simulink model "Assignment2_6"  (R2021b)
settings: Solver=ode45  StartTime=0.0  StopTime=0.1  RelTol=1e-3
libraries: eeGeneralControl x12, spsGroundLib x6, spsSeriesRLCBranchLib x6, spsBreakerLib x5, spsCurrentMeasurementLib x4, spsSeriesRLCLoadLib x3, spsACVoltageSourceLib x2, spspowerguiLib x1
settings Model: Creator=yyx  LastModifiedBy=Divin

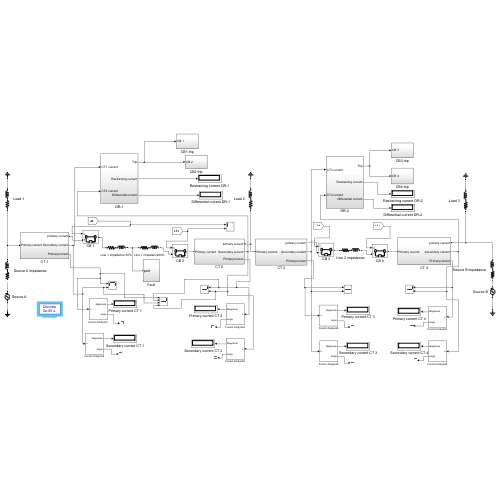
[thumbnail: Simulink's stored preview of the top-level diagram]
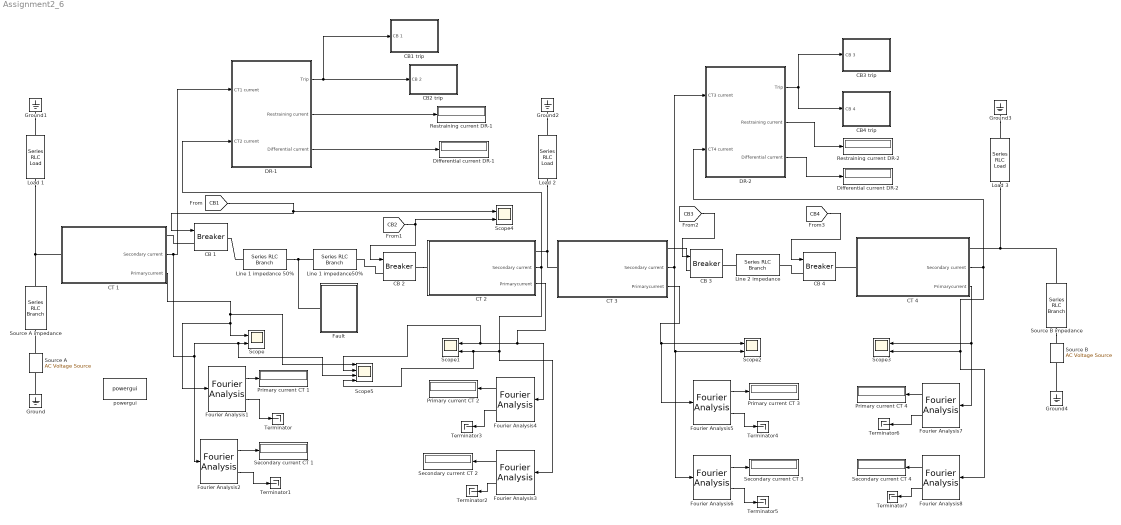
== system Assignment2_6 ==
  CB {1..4} (4 alike) : spsBreakerLib/Breaker  InitialState=1  SwitchingTimes="[1/60  5/60]"  External=on  BreakerResistance=0.01  SnubberResistance=1e6  SnubberCapacitance=inf  Measurements=None  MoreParameters=on  NoBreakLoop=off
      settings: SourceProductBaseCode=PS
  CB1 trip : Subsystem
  CB2 trip : Subsystem
  CB3 trip : Subsystem
  CB4 trip : Subsystem
  CT 1 : Subsystem
      settings: PortSchema="{\"entries\":[{\"content\":{\"sides\":[{\"content\":{\"connectorIds\":[\"LConn1\"]},\"type\":\"ConnectorPlacement.EquallySpacedRectSide\",\"uuid\":\"b6c390a4-07fb-4b4f-8c93-5dabcb0efae7\"},{\"content\":{\"connectorIds\":[\"RConn1\",\"Out1\",\"Out2\"],\"side\":\"RIGHT\"},\"type\":\"ConnectorPlacement.EquallySpacedRectSide\",\"uuid\":\"a4be9a2e-9ce7-48b9-b5c8-de816166e0f8\"},{\"content\":{\"connectorIds\":[],\"side\":\"TOP\"},\"type\":\"ConnectorPlacement.EquallySpacedRectSide\",\"uuid\":\"65e6e7fb-be75-4aba-a80b-3e233021d29a\"},{\"content\":{\"connectorIds\":[],\"side\":\"BOTTOM\"},\"type\":\"ConnectorPlacement.EquallySpacedRectSide\",\"uuid\":\"e137e53f-9924-4e8e-9c53-452c54d47921\"}]},\"type\":\"ConnectorPlacement.EquallySpacedConnector\",\"uuid\":\"c098d5a2-c3b9-46e4-a182-de1093aeec0c\"}],\"packageUris\":[\"http://schema.mathworks.com/mf0/Connector/R2020b\"],\"version\":\"1.0\"}"
  CT 2 : Subsystem
      settings: PortSchema="{\"entries\":[{\"content\":{\"sides\":[{\"content\":{\"connectorIds\":[\"LConn1\"]},\"type\":\"ConnectorPlacement.EquallySpacedRectSide\",\"uuid\":\"b6c390a4-07fb-4b4f-8c93-5dabcb0efae7\"},{\"content\":{\"connectorIds\":[\"RConn1\",\"Out1\",\"Out2\"],\"side\":\"RIGHT\"},\"type\":\"ConnectorPlacement.EquallySpacedRectSide\",\"uuid\":\"a4be9a2e-9ce7-48b9-b5c8-de816166e0f8\"},{\"content\":{\"connectorIds\":[],\"side\":\"TOP\"},\"type\":\"ConnectorPlacement.EquallySpacedRectSide\",\"uuid\":\"65e6e7fb-be75-4aba-a80b-3e233021d29a\"}]},\"type\":\"ConnectorPlacement.EquallySpacedConnector\",\"uuid\":\"c098d5a2-c3b9-46e4-a182-de1093aeec0c\"}],\"packageUris\":[\"http://schema.mathworks.com/mf0/Connector/R2020b\"],\"version\":\"1.0\"}"
  CT 3 : Subsystem
      settings: PortSchema="{\"entries\":[{\"content\":{\"sides\":[{\"content\":{\"connectorIds\":[\"LConn1\"]},\"type\":\"ConnectorPlacement.EquallySpacedRectSide\",\"uuid\":\"b6c390a4-07fb-4b4f-8c93-5dabcb0efae7\"},{\"content\":{\"connectorIds\":[\"RConn1\",\"Out1\",\"Out2\"],\"side\":\"RIGHT\"},\"type\":\"ConnectorPlacement.EquallySpacedRectSide\",\"uuid\":\"a4be9a2e-9ce7-48b9-b5c8-de816166e0f8\"},{\"content\":{\"connectorIds\":[],\"side\":\"TOP\"},\"type\":\"ConnectorPlacement.EquallySpacedRectSide\",\"uuid\":\"65e6e7fb-be75-4aba-a80b-3e233021d29a\"}]},\"type\":\"ConnectorPlacement.EquallySpacedConnector\",\"uuid\":\"c098d5a2-c3b9-46e4-a182-de1093aeec0c\"}],\"packageUris\":[\"http://schema.mathworks.com/mf0/Connector/R2020b\"],\"version\":\"1.0\"}"
  CT 4 : Subsystem
      settings: PortSchema="{\"entries\":[{\"content\":{\"sides\":[{\"content\":{\"connectorIds\":[\"LConn1\"]},\"type\":\"ConnectorPlacement.EquallySpacedRectSide\",\"uuid\":\"b6c390a4-07fb-4b4f-8c93-5dabcb0efae7\"},{\"content\":{\"connectorIds\":[\"RConn1\",\"Out1\",\"Out2\"],\"side\":\"RIGHT\"},\"type\":\"ConnectorPlacement.EquallySpacedRectSide\",\"uuid\":\"a4be9a2e-9ce7-48b9-b5c8-de816166e0f8\"},{\"content\":{\"connectorIds\":[],\"side\":\"TOP\"},\"type\":\"ConnectorPlacement.EquallySpacedRectSide\",\"uuid\":\"65e6e7fb-be75-4aba-a80b-3e233021d29a\"},{\"content\":{\"connectorIds\":[],\"side\":\"BOTTOM\"},\"type\":\"ConnectorPlacement.EquallySpacedRectSide\",\"uuid\":\"ae0a5bc8-40b7-4a3b-a403-59123a5fd983\"}]},\"type\":\"ConnectorPlacement.EquallySpacedConnector\",\"uuid\":\"c098d5a2-c3b9-46e4-a182-de1093aeec0c\"}],\"packageUris\":[\"http://schema.mathworks.com/mf0/Connector/R2020b\"],\"version\":\"1.0\"}"
  DR-1 : Subsystem
  DR-2 : Subsystem
  Differential current DR-1 : Display
  Differential current DR-2 : Display
  Fault : Subsystem
  Fourier Analysis{1..8} (8 alike) : eeGeneralControl/Fourier Analysis  f=60  n=[1]  M0=0  Ph0=0  BufferSize=8192  Ts=0
      settings: SourceProductBaseCode=PS
  Ground{,1..4} (5 alike) : spsGroundLib/Ground  LConnTagsString=a
  Line 1 impedance 50% : spsSeriesRLCBranchLib/Series RLC Branch  LConnTagsString=__new0  RConnTagsString=__new0  BranchType=RL  Resistance=1  Inductance=0.026525  SetiL0=off  InitialCurrent=0  Capacitance=1e-6  Setx0=off  InitialVoltage=0  Measurements=None
  Line 1 impedance50% : spsSeriesRLCBranchLib/Series RLC Branch  LConnTagsString=__new0  RConnTagsString=__new0  BranchType=RL  Resistance=1  Inductance=0.026525  SetiL0=off  InitialCurrent=0  Capacitance=1e-6  Setx0=off  InitialVoltage=0  Measurements=None
  Line 2 impedance : spsSeriesRLCBranchLib/Series RLC Branch  LConnTagsString=__new0  RConnTagsString=__new0  BranchType=RL  Resistance=2  Inductance=0.05305  SetiL0=off  InitialCurrent=0  Capacitance=1e-6  Setx0=off  InitialVoltage=0  Measurements=None
  Load 1 : spsSeriesRLCLoadLib/Series RLC Load  LConnTagsString=a  RConnTagsString=__new0  NominalVoltage=138000  NominalFrequency=60  ActivePower=100e6  InductivePower=30e6  CapacitivePower=0  Setx0=off  InitialVoltage=0  SetiL0=off  InitialCurrent=0  Measurements=None  LoadType=constant Z
  Load 2 : spsSeriesRLCLoadLib/Series RLC Load  LConnTagsString=a  RConnTagsString=__new0  NominalVoltage=138000  NominalFrequency=60  ActivePower=100e6  InductivePower=30e6  CapacitivePower=0  Setx0=off  InitialVoltage=0  SetiL0=off  InitialCurrent=0  Measurements=None  LoadType=constant Z
  Load 3 : spsSeriesRLCLoadLib/Series RLC Load  LConnTagsString=a  RConnTagsString=__new0  NominalVoltage=138000  NominalFrequency=60  ActivePower=100e6  InductivePower=30e6  CapacitivePower=0  Setx0=off  InitialVoltage=0  SetiL0=off  InitialCurrent=0  Measurements=None  LoadType=constant Z
  Primary current CT {1..4} (4 alike) : Display
  Restraining current DR-1 : Display
  Restraining current DR-2 : Display
  Scope{,1..4} (5 alike) : Scope  NumInputPorts=2
  Scope5 : Scope  NumInputPorts=4
  Secondary current CT {1..4} (4 alike) : Display
  Source A : spsACVoltageSourceLib/AC Voltage Source  Amplitude=158000  Phase=0  Frequency=60  SampleTime=0  Measurements=None  BusType=swing  Pref=10e3  Qref=0  Qmin=-inf  Qmax=+inf
  Source A impedance : spsSeriesRLCBranchLib/Series RLC Branch  LConnTagsString=__new0  RConnTagsString=__new0  BranchType=RL  Resistance=1  Inductance=0.02653  SetiL0=off  InitialCurrent=0  Capacitance=1e-6  Setx0=off  InitialVoltage=0  Measurements=None
  Source B : spsACVoltageSourceLib/AC Voltage Source  Amplitude=157000  Phase=-15  Frequency=60  SampleTime=0  Measurements=None  BusType=swing  Pref=10e3  Qref=0  Qmin=-inf  Qmax=+inf
  Source B impedance : spsSeriesRLCBranchLib/Series RLC Branch  LConnTagsString=__new0  RConnTagsString=__new0  BranchType=RL  Resistance=1  Inductance=0.02653  SetiL0=off  InitialCurrent=0  Capacitance=1e-6  Setx0=off  InitialVoltage=0  Measurements=None
  Terminator{,1..7} (8 alike) : Terminator
  powergui : spspowerguiLib/powergui  Priority=1  SimulationMode=Discrete  SampleTime=50e-6  frequency=60  Iterations=50  frequencyindice=0  Pbase=100e6  ErrMax=1e-4  UnitsV=kV  UnitsW=MW  buscounter=0  FunctionMessages=off  echomessages=off  EnableUseOfTLC=off  CurrentSourceSwitches=off  DisableSnubberDevices=off  DisableRonSwitches=off  DisableVfSwitches=off  DisplayEquations=off  AutomaticDiscreteSolvers=off  SolverType=Tustin/Backward Euler (TBE)  Interpol=off  ExternalGateDelay=off  methode=off  Ts=100  x0status=blocks  SPID=on  SwTol=0  HookPort=off  NonlinearTolerance=1e-4  nMaxIteration=100  ContinueOnMaxIteration=off  RestoreLinks=warning  ResistiveCurrentMeasurement=off  Frange=[0:2:500]  Ylog=off  Xlog=on  ShowGrid=off  save=off  variable=ZData  structure=0  ZoomFFT=off  StartTime=0.0  cycles=1  DisplayStyle=1  fundamental=60  FreqAxis=off  MaxFrequency=1000  frequencyindicesteady=1  RmsSteady=1  display=off
  wires:
  CT 2/1(Secondary current) -> Fourier Analysis3/1, Scope5/4, Scope1/2, DR-1/2(CT2 current)
  DR-1/1(Trip) -> CB2 trip/1(CB 2), CB1 trip/1(CB 1)
  [CB2] -> Scope4/2, CB 2/1
  CT 1/1(Secondary current) -> DR-1/1(CT1 current), Fourier Analysis2/1, Scope5/3, Scope/2
  CT 1/2(Primarycurrent) -> Scope5/1, Scope/1, Fourier Analysis1/1
  CT 3/1(Secondary current) -> DR-2/1(CT3 current), Fourier Analysis6/1, Scope2/2
  CT 4/1(Secondary current) -> Fourier Analysis8/1, Scope3/2, DR-2/2(CT4 current)
  DR-2/1(Trip) -> CB4 trip/1(CB 4), CB3 trip/1(CB 3)
  [CB3] -> CB 3/1
  [CB4] -> CB 4/1
  CT 2/2(Primarycurrent) -> Fourier Analysis4/1, Scope5/2, Scope1/1
  CT 3/2(Primarycurrent) -> Fourier Analysis5/1, Scope2/1
  CT 4/2(Primarycurrent) -> Scope3/1, Fourier Analysis7/1
  Fourier Analysis1/1 -> Primary current CT 1/1
  Fourier Analysis1/2 -> Terminator/1
  Fourier Analysis2/2 -> Terminator1/1
  Fourier Analysis2/1 -> Secondary current CT 1/1
  Fourier Analysis3/2 -> Terminator2/1
  Fourier Analysis3/1 -> Secondary current CT 2/1
  Fourier Analysis4/2 -> Terminator3/1
  Fourier Analysis4/1 -> Primary current CT 2/1
  Fourier Analysis5/2 -> Terminator4/1
  Fourier Analysis5/1 -> Primary current CT 3/1
  Fourier Analysis6/2 -> Terminator5/1
  Fourier Analysis6/1 -> Secondary current CT 3/1
  Fourier Analysis7/2 -> Terminator6/1
  Fourier Analysis7/1 -> Primary current CT 4/1
  Fourier Analysis8/2 -> Terminator7/1
  Fourier Analysis8/1 -> Secondary current CT 4/1
  DR-1/2(Restraining current) -> Restraining current DR-1/1
  DR-1/3(Differential current) -> Differential current DR-1/1
  DR-2/2(Restraining current) -> Restraining current DR-2/1
  DR-2/3(Differential current) -> Differential current DR-2/1
  [CB1] -> CB 1/1, Scope4/1
  connections:
  Ground/LConn1 -- Source A/LConn1
  Source A impedance/RConn1 -- Load 1/LConn1 -- CT 1/LConn1
  Ground1/LConn1 -- Load 1/RConn1
  CB 1/LConn1 -- CT 1/RConn1
  Ground2/LConn1 -- Load 2/RConn1
  Load 2/LConn1 -- CT 3/LConn1 -- CT 2/RConn1
  CT 3/RConn1 -- CB 3/LConn1
  Line 2 impedance/LConn1 -- CB 3/RConn1
  CB 4/LConn1 -- Line 2 impedance/RConn1
  CT 4/LConn1 -- CB 4/RConn1
  Ground3/LConn1 -- Load 3/RConn1
  Load 3/LConn1 -- Source B impedance/RConn1 -- CT 4/RConn1
  Source B impedance/LConn1 -- Source B/RConn1
  Ground4/LConn1 -- Source B/LConn1
  CB 2/LConn1 -- Line 1 impedance50%/RConn1
  CB 2/RConn1 -- CT 2/LConn1
  Line 1 impedance 50%/LConn1 -- CB 1/RConn1
  Line 1 impedance 50%/RConn1 -- Fault/LConn1 -- Line 1 impedance50%/LConn1
  Source A/RConn1 -- Source A impedance/LConn1

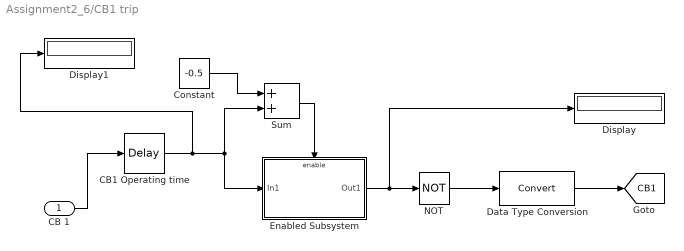
== system Assignment2_6/CB1 trip ==
  CB 1 : Inport
  CB1 Operating time : TransportDelay  DelayTime=15e-3
  Constant : Constant  Value=-0.5
  Data Type Conversion : DataTypeConversion
  Display : Display
  Display1 : Display
  Enabled Subsystem : Subsystem  TreatAsAtomicUnit=on
  NOT : Logic  Operator=NOT  IconShape=distinctive  AllPortsSameDT=off  OutDataTypeStr=boolean
  Sum : Sum
  tag scope: CB1=global
  wires:
  Sum/1 -> Enabled Subsystem/Enable
  CB 1/1 -> CB1 Operating time/1
  Constant/1 -> Sum/1
  CB1 Operating time/1 -> Display1/1, Sum/2, Enabled Subsystem/1(In1)
  Enabled Subsystem/1(Out1) -> Display/1, NOT/1
  NOT/1 -> Data Type Conversion/1
  Data Type Conversion/1 -> [CB1]

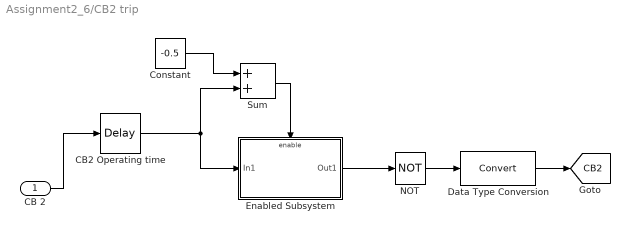
== system Assignment2_6/CB2 trip ==
  CB 2 : Inport
  CB2 Operating time : TransportDelay  DelayTime=25e-3
  Constant : Constant  Value=-0.5
  Data Type Conversion : DataTypeConversion
  Enabled Subsystem : Subsystem  TreatAsAtomicUnit=on
  NOT : Logic  Operator=NOT  IconShape=distinctive  AllPortsSameDT=off  OutDataTypeStr=boolean
  Sum : Sum
  tag scope: CB2=global
  wires:
  Sum/1 -> Enabled Subsystem/Enable
  CB 2/1 -> CB2 Operating time/1
  Constant/1 -> Sum/1
  CB2 Operating time/1 -> Sum/2, Enabled Subsystem/1(In1)
  Enabled Subsystem/1(Out1) -> NOT/1
  NOT/1 -> Data Type Conversion/1
  Data Type Conversion/1 -> [CB2]

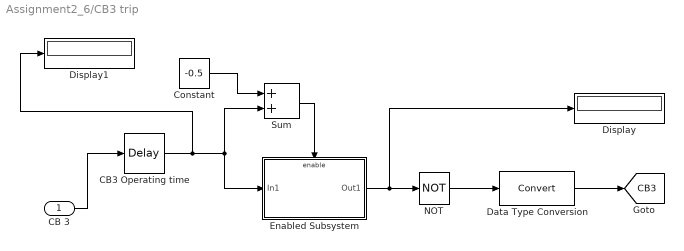
== system Assignment2_6/CB3 trip ==
  CB 3 : Inport
  CB3 Operating time : TransportDelay  DelayTime=18e-3
  Constant : Constant  Value=-0.5
  Data Type Conversion : DataTypeConversion
  Display : Display
  Display1 : Display
  Enabled Subsystem : Subsystem  TreatAsAtomicUnit=on
  NOT : Logic  Operator=NOT  IconShape=distinctive  AllPortsSameDT=off  OutDataTypeStr=boolean
  Sum : Sum
  tag scope: CB3=global
  wires:
  Sum/1 -> Enabled Subsystem/Enable
  CB 3/1 -> CB3 Operating time/1
  Constant/1 -> Sum/1
  CB3 Operating time/1 -> Display1/1, Sum/2, Enabled Subsystem/1(In1)
  Enabled Subsystem/1(Out1) -> Display/1, NOT/1
  NOT/1 -> Data Type Conversion/1
  Data Type Conversion/1 -> [CB3]

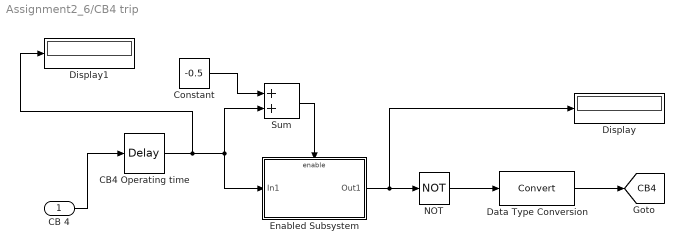
== system Assignment2_6/CB4 trip ==
  CB 4 : Inport
  CB4 Operating time : TransportDelay  DelayTime=21e-3
  Constant : Constant  Value=-0.5
  Data Type Conversion : DataTypeConversion
  Display : Display
  Display1 : Display
  Enabled Subsystem : Subsystem  TreatAsAtomicUnit=on
  NOT : Logic  Operator=NOT  IconShape=distinctive  AllPortsSameDT=off  OutDataTypeStr=boolean
  Sum : Sum
  tag scope: CB4=global
  wires:
  Sum/1 -> Enabled Subsystem/Enable
  CB 4/1 -> CB4 Operating time/1
  Constant/1 -> Sum/1
  CB4 Operating time/1 -> Display1/1, Sum/2, Enabled Subsystem/1(In1)
  Enabled Subsystem/1(Out1) -> Display/1, NOT/1
  NOT/1 -> Data Type Conversion/1
  Data Type Conversion/1 -> [CB4]

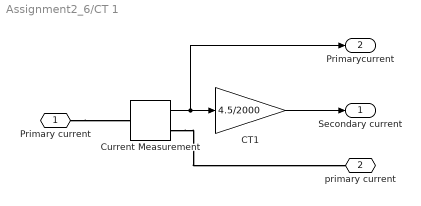
== system Assignment2_6/CT 1 ==
  CT1 : Gain  Gain=4.5/2000
  Current Measurement : spsCurrentMeasurementLib/Current Measurement  PhasorSimulation=off  OutputType=Complex  PSBequivalent=0
  Primary current : PMIOPort  Side=Left
  primary current : PMIOPort  Port=2  Side=Right
  Secondary current : Outport
  Primarycurrent : Outport  Port=2
  wires:
  Current Measurement/1 -> Primarycurrent/1, CT1/1
  CT1/1 -> Secondary current/1
  connections:
  Primary current/RConn1 -- Current Measurement/LConn1
  Current Measurement/RConn1 -- primary current/RConn1

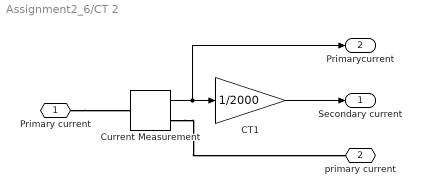
== system Assignment2_6/CT 2 ==
  CT1 : Gain  Gain=1/2000
  Current Measurement : spsCurrentMeasurementLib/Current Measurement  PhasorSimulation=off  OutputType=Complex  PSBequivalent=0
  Primary current : PMIOPort  Side=Left
  primary current : PMIOPort  Port=2  Side=Right
  Secondary current : Outport
  Primarycurrent : Outport  Port=2
  wires:
  CT1/1 -> Secondary current/1
  Current Measurement/1 -> Primarycurrent/1, CT1/1
  connections:
  Primary current/RConn1 -- Current Measurement/LConn1
  Current Measurement/RConn1 -- primary current/RConn1

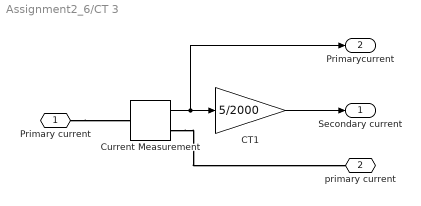
== system Assignment2_6/CT 3 ==
  CT1 : Gain  Gain=5/2000
  Current Measurement : spsCurrentMeasurementLib/Current Measurement  PhasorSimulation=off  OutputType=Complex  PSBequivalent=0
  Primary current : PMIOPort  Side=Left
  primary current : PMIOPort  Port=2  Side=Right
  Secondary current : Outport
  Primarycurrent : Outport  Port=2
  wires:
  Current Measurement/1 -> Primarycurrent/1, CT1/1
  CT1/1 -> Secondary current/1
  connections:
  Primary current/RConn1 -- Current Measurement/LConn1
  Current Measurement/RConn1 -- primary current/RConn1

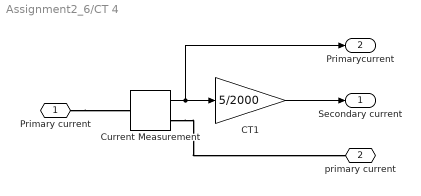
== system Assignment2_6/CT 4 ==
  CT1 : Gain  Gain=5/2000
  Current Measurement : spsCurrentMeasurementLib/Current Measurement  PhasorSimulation=off  OutputType=Complex  PSBequivalent=0
  Primary current : PMIOPort  Side=Left
  primary current : PMIOPort  Port=2  Side=Right
  Secondary current : Outport
  Primarycurrent : Outport  Port=2
  wires:
  Current Measurement/1 -> Primarycurrent/1, CT1/1
  CT1/1 -> Secondary current/1
  connections:
  Primary current/RConn1 -- Current Measurement/LConn1
  Current Measurement/RConn1 -- primary current/RConn1

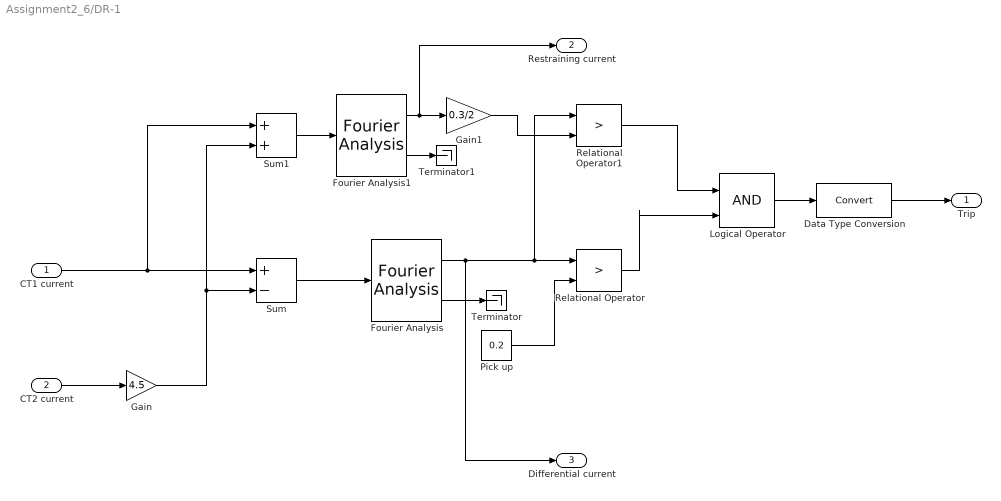
== system Assignment2_6/DR-1 ==
  CT1 current : Inport
  CT2 current : Inport  Port=2
  Data Type Conversion : DataTypeConversion
  Fourier Analysis : eeGeneralControl/Fourier Analysis  f=60  n=[1]  M0=0  Ph0=0  BufferSize=8192  Ts=0
      settings: SourceProductBaseCode=PS
  Fourier Analysis1 : eeGeneralControl/Fourier Analysis  f=60  n=[1]  M0=0  Ph0=0  BufferSize=8192  Ts=0
      settings: SourceProductBaseCode=PS
  Gain : Gain  Gain=4.5
  Gain1 : Gain  Gain=0.3/2
  Logical Operator : Logic  IconShape=distinctive  AllPortsSameDT=off  OutDataTypeStr=boolean
  Pick up : Constant  Value=0.2
  Relational Operator : RelationalOperator  Operator=>  OutDataTypeStr=boolean  RndMeth=Simplest
  Relational Operator1 : RelationalOperator  Operator=>  OutDataTypeStr=boolean  RndMeth=Simplest
  Sum : Sum  Inputs=+-
  Sum1 : Sum
  Terminator : Terminator
  Terminator1 : Terminator
  Trip : Outport
  Restraining current : Outport  Port=2
  Differential current : Outport  Port=3
  wires:
  CT1 current/1 -> Sum1/1, Sum/1
  Fourier Analysis/2 -> Terminator/1
  Fourier Analysis/1 -> Relational Operator1/1, Relational Operator/1, Differential current/1
  Pick up/1 -> Relational Operator/2
  Sum/1 -> Fourier Analysis/1
  Data Type Conversion/1 -> Trip/1
  Fourier Analysis1/2 -> Terminator1/1
  Relational Operator1/1 -> Logical Operator/1
  Logical Operator/1 -> Data Type Conversion/1
  Relational Operator/1 -> Logical Operator/2
  Sum1/1 -> Fourier Analysis1/1
  Fourier Analysis1/1 -> Gain1/1, Restraining current/1
  Gain1/1 -> Relational Operator1/2
  CT2 current/1 -> Gain/1
  Gain/1 -> Sum/2, Sum1/2

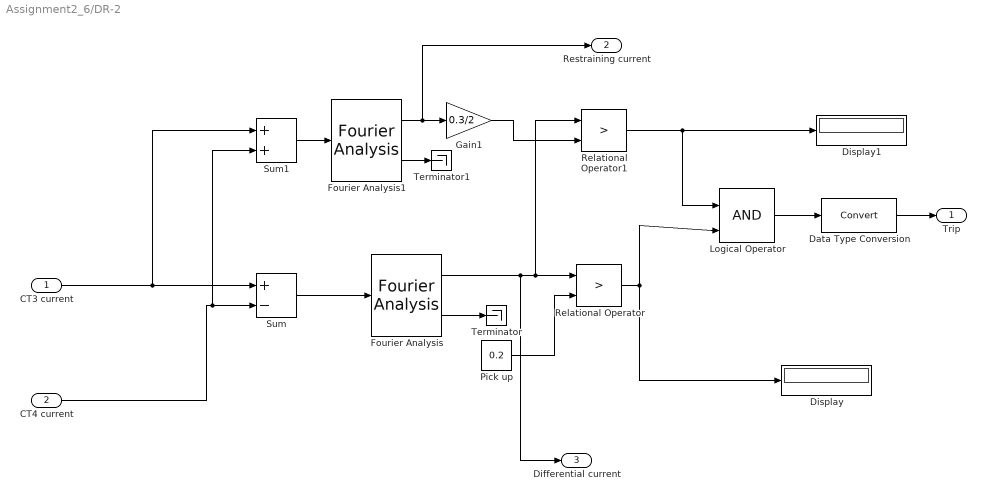
== system Assignment2_6/DR-2 ==
  CT3 current : Inport
  CT4 current : Inport  Port=2
  Data Type Conversion : DataTypeConversion
  Display : Display
  Display1 : Display
  Fourier Analysis : eeGeneralControl/Fourier Analysis  f=60  n=[1]  M0=0  Ph0=0  BufferSize=8192  Ts=0
      settings: SourceProductBaseCode=PS
  Fourier Analysis1 : eeGeneralControl/Fourier Analysis  f=60  n=[1]  M0=0  Ph0=0  BufferSize=8192  Ts=0
      settings: SourceProductBaseCode=PS
  Gain1 : Gain  Gain=0.3/2
  Logical Operator : Logic  IconShape=distinctive  AllPortsSameDT=off  OutDataTypeStr=boolean
  Pick up : Constant  Value=0.2
  Relational Operator : RelationalOperator  Operator=>  OutDataTypeStr=boolean  RndMeth=Simplest
  Relational Operator1 : RelationalOperator  Operator=>  OutDataTypeStr=boolean  RndMeth=Simplest
  Sum : Sum  Inputs=+-
  Sum1 : Sum
  Terminator : Terminator
  Terminator1 : Terminator
  Trip : Outport
  Restraining current : Outport  Port=2
  Differential current : Outport  Port=3
  wires:
  Fourier Analysis/2 -> Terminator/1
  Pick up/1 -> Relational Operator/2
  Sum/1 -> Fourier Analysis/1
  Relational Operator/1 -> Logical Operator/2, Display/1
  Data Type Conversion/1 -> Trip/1
  Fourier Analysis/1 -> Differential current/1, Relational Operator1/1, Relational Operator/1
  CT3 current/1 -> Sum1/1, Sum/1
  Relational Operator1/1 -> Logical Operator/1, Display1/1
  CT4 current/1 -> Sum1/2, Sum/2
  Fourier Analysis1/2 -> Terminator1/1
  Logical Operator/1 -> Data Type Conversion/1
  Sum1/1 -> Fourier Analysis1/1
  Fourier Analysis1/1 -> Restraining current/1, Gain1/1
  Gain1/1 -> Relational Operator1/2

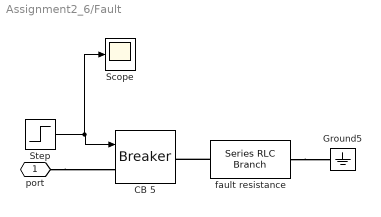
== system Assignment2_6/Fault ==
  CB 5 : spsBreakerLib/Breaker  InitialState=0  SwitchingTimes="[0.01  0.03]"  External=on  BreakerResistance=0.01  SnubberResistance=1e6  SnubberCapacitance=inf  Measurements=None  MoreParameters=on  NoBreakLoop=off
      settings: SourceProductBaseCode=PS
  Ground5 : spsGroundLib/Ground  LConnTagsString=a
  Scope : Scope
  Step : Step  Time=20e-3  SampleTime=0
  fault resistance : spsSeriesRLCBranchLib/Series RLC Branch  LConnTagsString=__new0  RConnTagsString=__new0  BranchType=R  Resistance=448.6  Inductance=0.026525  SetiL0=off  InitialCurrent=0  Capacitance=1e-6  Setx0=off  InitialVoltage=0  Measurements=None
  port : PMIOPort  Side=Left
  wires:
  Step/1 -> Scope/1, CB 5/1
  connections:
  port/RConn1 -- CB 5/LConn1
  fault resistance/LConn1 -- CB 5/RConn1
  fault resistance/RConn1 -- Ground5/LConn1

== system Assignment2_6/CB1 trip/Enabled Subsystem ==
  In1 : Inport
  Enable : EnablePort
  Out1 : Outport
  wires:
  In1/1 -> Out1/1

== system Assignment2_6/CB2 trip/Enabled Subsystem ==
  In1 : Inport
  Enable : EnablePort
  Out1 : Outport
  wires:
  In1/1 -> Out1/1

== system Assignment2_6/CB3 trip/Enabled Subsystem ==
  In1 : Inport
  Enable : EnablePort
  Out1 : Outport
  wires:
  In1/1 -> Out1/1

== system Assignment2_6/CB4 trip/Enabled Subsystem ==
  In1 : Inport
  Enable : EnablePort
  Out1 : Outport
  wires:
  In1/1 -> Out1/1
